simulink model "GEB"  (R2020a)
settings: Solver=FixedStepAuto  StartTime=0  StopTime=1  FixedStep=1  RelTol=1e-3
settings Model: Creator=Aaron  LastModifiedBy=Aaron

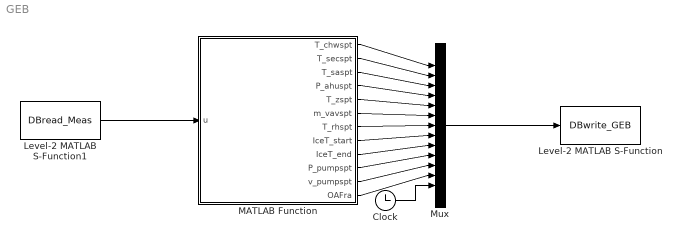
== system GEB ==
  Clock : Clock
  Level-2 MATLAB S-Function : M-S-Function  FunctionName=DBwrite_GEB
  Level-2 MATLAB S-Function1 : M-S-Function  FunctionName=DBread_Meas
  MATLAB Function : MATLAB Function  TreatAsAtomicUnit=on
  Mux : Mux  Inputs=13
  wires:
  Clock/1 -> Mux/13
  Mux/1 -> Level-2 MATLAB S-Function/1
  MATLAB Function/1(T_chwspt) -> Mux/1
  MATLAB Function/2(T_secspt) -> Mux/2
  MATLAB Function/4(P_ahuspt) -> Mux/4
  MATLAB Function/3(T_saspt) -> Mux/3
  MATLAB Function/5(T_zspt) -> Mux/5
  MATLAB Function/7(T_rhspt) -> Mux/7
  MATLAB Function/6(m_vavspt) -> Mux/6
  MATLAB Function/8(IceT_start) -> Mux/8
  MATLAB Function/9(IceT_end) -> Mux/9
  MATLAB Function/10(P_pumpspt) -> Mux/10
  MATLAB Function/11(v_pumpspt) -> Mux/11
  MATLAB Function/12(OAFra) -> Mux/12
  Level-2 MATLAB S-Function1/1 -> MATLAB Function/1(u)

== matlab function GEB/MATLAB Function ==
  data: T_chwspt output; u input; T_secspt output; T_saspt output; P_ahuspt output; T_zspt output; m_vavspt output; T_rhspt output; IceT_start output; IceT_end output; P_pumpspt output; v_pumpspt output; OAFra output
function [T_chwspt,T_secspt,T_saspt,P_ahuspt,T_zspt,m_vavspt,...
    T_rhspt,IceT_start,IceT_end,P_pumpspt,v_pumpspt,OAFra] = fcn(u)
pause(20);
T_chwspt=4;
T_secspt=7;
T_saspt=12;
P_ahuspt=1.5;
T_zspt=24;
m_vavspt=0.12;
T_rhspt=u(1,4);
IceT_start=15*10*60;
IceT_end=15*30*60;
P_pumpspt=20;
v_pumpspt=36;
OAFra=0.4;
